simulink model "DETUMBLE_POINTING"  (R2025b)
settings: Solver=ode45  StartTime=0.0  StopTime=5  RelTol=1e-3
undefined symbols (not defined in the file): J, J_rotor, J_satelit, Jw, Kd, Kd_detumble, Kp, omega0, omega_high, omega_low, omega_w0, theta0, theta_ref
settings Model: Creator=bbtp  LastModifiedBy=bbtp
settings SolverCC: ZeroCrossAlgorithm=Adaptive
settings DebuggingCC: IgnoredZcDiagnostic=none

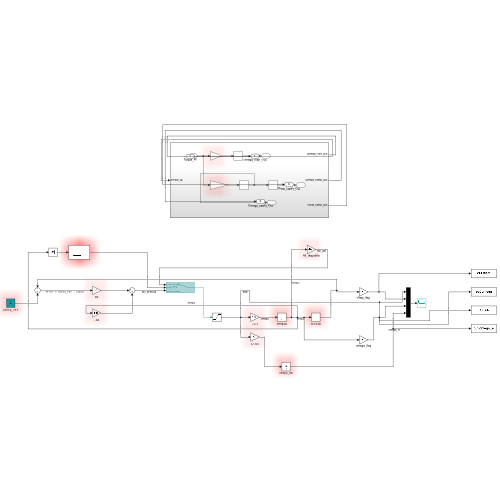
[thumbnail: Simulink's stored preview of the top-level diagram]
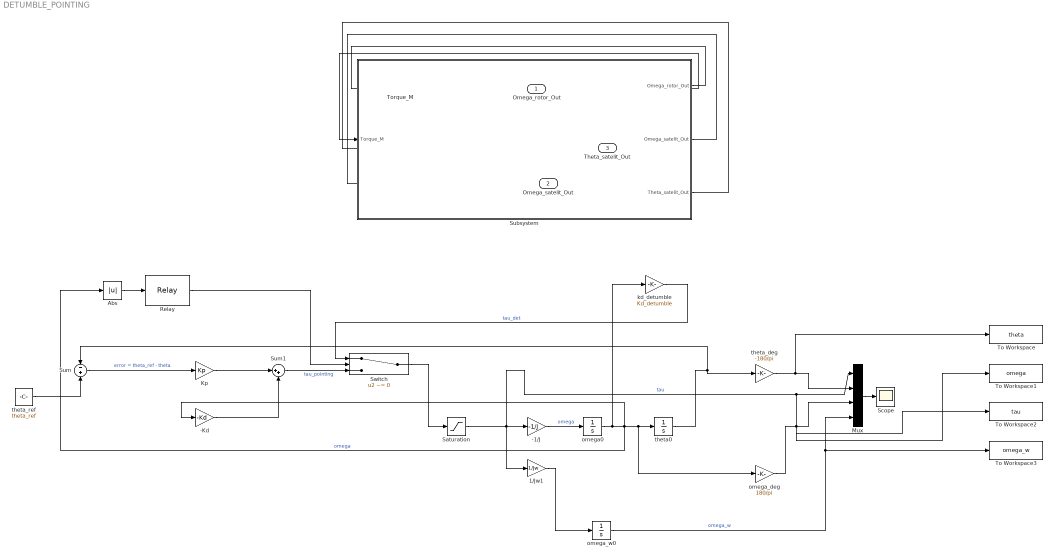
== system DETUMBLE_POINTING ==
  Torque_M : Inport
  -1/J : Gain  Gain=-1/J
  -Kd : Gain  Gain=-Kd
  1/Jw1 : Gain  Gain=1/Jw
  Abs : Abs  SaturateOnIntegerOverflow=off
  Kp : Gain  Gain=Kp
  Mux : Mux
  Relay : Relay  OnSwitchValue=omega_high  OffSwitchValue=omega_low
  Saturation : Saturate
  Scope : Scope
      settings: ActiveDisplayYMinimum=-411567.73029706057  ActiveDisplayYMaximum=343540.60888628056
  Subsystem : Subsystem
  Sum : Sum  Inputs=-+
  Sum1 : Sum  Inputs=|++
  Switch : Switch  Criteria=u2 ~= 0  SaturateOnIntegerOverflow=off  InputSameDT=off
  To Workspace : ToWorkspace  VariableName=theta  SaveFormat=Timeseries  SampleTime=-1
  To Workspace1 : ToWorkspace  VariableName=omega  SaveFormat=Timeseries  SampleTime=-1
  To Workspace2 : ToWorkspace  VariableName=tau  SaveFormat=Timeseries  SampleTime=-1
  To Workspace3 : ToWorkspace  VariableName=omega_w  SaveFormat=Timeseries  SampleTime=-1
  kd_detumble : Gain  Gain=Kd_detumble
  omega0 : Integrator  InitialCondition=omega0
  omega_deg : Gain  Gain=180/pi
  omega_w0 : Integrator  InitialCondition=omega_w0
  theta0 : Integrator  InitialCondition=-theta0
  theta_deg : Gain  Gain=-180/pi
  theta_ref : Constant  Value=theta_ref
  Omega_rotor_Out : Outport
  Omega_satelit_Out : Outport  Port=2
  Theta_satelit_Out : Outport  Port=3
  wires:
  Mux/1 -> Scope/1
  -Kd/1 -> Sum1/2
  theta0/1 -> Sum/1, theta_deg/1
  omega_deg/1 -> To Workspace1/1, Mux/3
  theta_ref/1 -> Sum/2
  theta_deg/1 -> To Workspace/1, Mux/2
  Kp/1 -> Sum1/1
  omega0/1 -> kd_detumble/1, Abs/1, -Kd/1, omega_deg/1, theta0/1  "omega"
  Saturation/1 -> 1/Jw1/1, To Workspace2/1, Mux/1, -1/J/1  "tau"
  Sum/1 -> Kp/1  "error = theta_ref - theta"
  Switch/1 -> Saturation/1
  kd_detumble/1 -> Switch/1  "tau_det"
  Sum1/1 -> Switch/3  "tau_pointing"
  Relay/1 -> Switch/2
  -1/J/1 -> omega0/1  "omega"
  1/Jw1/1 -> omega_w0/1
  omega_w0/1 -> To Workspace3/1, Mux/4  "omega_w"
  Abs/1 -> Relay/1
  Torque_M/1 -> Subsystem/1(Torque_M)
  Subsystem/1(Omega_rotor_Out) -> Omega_rotor_Out/1
  Subsystem/2(Omega_satelit_Out) -> Omega_satelit_Out/1
  Subsystem/3(Theta_satelit_Out) -> Theta_satelit_Out/1

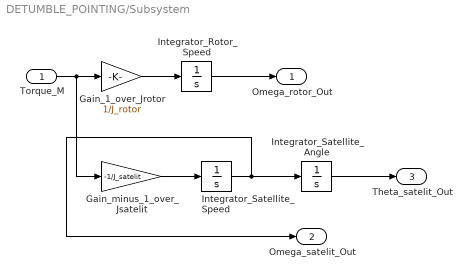
== system DETUMBLE_POINTING/Subsystem ==
  Torque_M : Inport
  Gain_1_over_Jrotor : Gain  Gain=1/J_rotor
  Gain_minus_1_over_Jsatelit : Gain  Gain=-1/J_satelit
  Integrator_Rotor_Speed : Integrator
  Integrator_Satellite_Angle : Integrator
  Integrator_Satellite_Speed : Integrator
  Omega_rotor_Out : Outport
  Omega_satelit_Out : Outport  Port=2
  Theta_satelit_Out : Outport  Port=3
  wires:
  Gain_1_over_Jrotor/1 -> Integrator_Rotor_Speed/1
  Integrator_Satellite_Speed/1 -> Omega_satelit_Out/1, Integrator_Satellite_Angle/1
  Integrator_Satellite_Angle/1 -> Theta_satelit_Out/1
  Torque_M/1 -> Gain_1_over_Jrotor/1, Gain_minus_1_over_Jsatelit/1
  Integrator_Rotor_Speed/1 -> Omega_rotor_Out/1
  Gain_minus_1_over_Jsatelit/1 -> Integrator_Satellite_Speed/1
